simulink model "Multibody_model_El_winch"  (R2023b)
settings: Solver=FixedStepAuto  StartTime=0.0  StopTime=25  FixedStep=0.001  RelTol=1e-3
model workspace (MATLAB code in the model file):
  | % Parameters
  | Q_max = 130; %L/min |  2 vales w max 65 L/min
  | 
  | %Load Parameters
  | m_pl = 1000;
  | r_d = 0.035;
  | ig = 5;
  | J_drum = 0.0006125; % 1/2MR^2
  | b_hat = 0.001;
  | 
  | % Motor Parameters
  | np=2;
  | P_N = 15000;
  | n_eff = 0.917;
  | n_rpm = 1469;
  | pf = 0.84;
  | I_N = 29;
  | Is_In = 8;
  | T_n = 97.5;
  | Ti_Tn = 3.1;
  | Tb_Tn = 3.6;
  | J_motor = 0.13;
  | 
  | % Inv-Gamma Circuit parameters
  | 
  | R_R_hat = 0.2052;
  | X_M_opt = 15.1061;
  | X_sig_opt = 0.3774;
  | omega_rN = 307.6666;
  | omega_N = 314.1593;
  | omega1 = omega_rN;
  | L_M_hat = X_M_opt/omega1;
  | L_sig_hat = X_sig_opt/omega1;
  | R_s = 0.619;
  | 
  | 
  | psi_ref = 20*P_N/(sqrt(2)*pi*np*I_N*n_rpm);
  | 
  | % Others
  | V_base = 400*sqrt(2)/sqrt(3);
  | I_max = I_N*3;
  | 
  | % Speed Controller
  | t_r = 1e-3;
  | w_BW = log(9)/t_r;
  | w_BWs = 0.1*w_BW;
  | J_hat = m_pl*((r_d/(ig))^2) + J_drum*((1/ig)^2) + J_motor;
  | kps = 2*J_hat*w_BWs/(3*np^2*psi_ref);
  | kis = w_BWs^2*2*J_hat/(3*np^2*psi_ref);
  | Ba = 2*J_hat/(3*np^2*psi_ref)*(w_BWs-b_hat/J_hat);
  | 
  | % Current Controller
  | kp = w_BW*L_sig_hat;
  | ki = w_BW^2*L_sig_hat;
  | Ra = w_BW*L_sig_hat - (R_R_hat + R_s);
  | R = R_R_hat + R_s;
undefined symbols (not defined in the file or in its folder): j, magnitude, X, Y, Z
libraries: sm_lib x44, fl_lib x24, nesl_utility x22, SimscapeFluids_lib x8, slpidlib x4, spsRMSLib x1, simulink x1
(part 3 of 4)

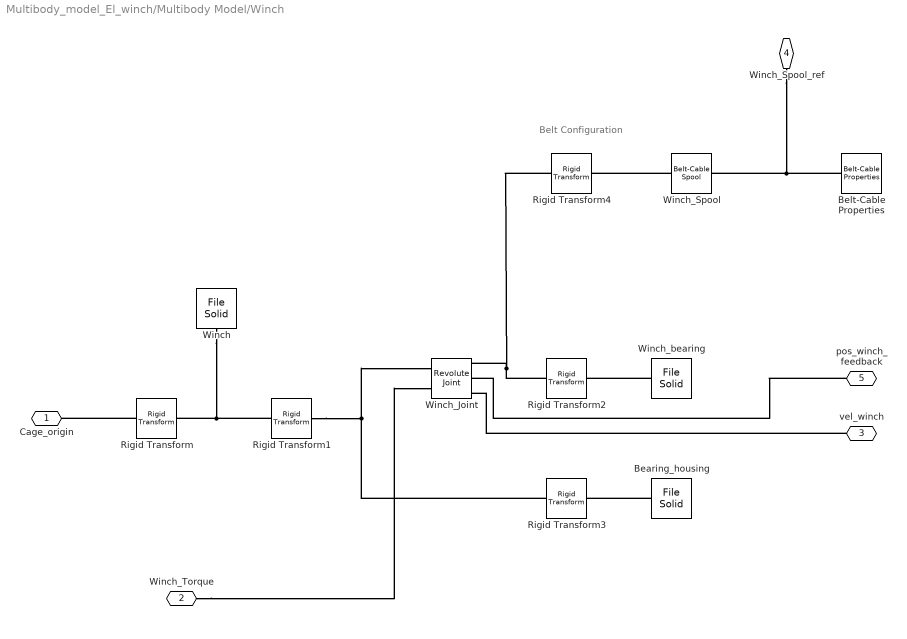
== system Multibody_model_El_winch/Multibody Model/Winch ==
  note: Belt Configuration
  Bearing_housing : sm_lib/Body Elements/File Solid  ExtGeomFileName=.\Parts_and_stl\Frame_connection_winch.STL  UnitType=Custom  ExtGeomFileUnits=mm  StepReaderType=HEX  ExportConvexHullGeometry=off  InertiaType=Custom  Mass=1  MassUnits=kg  CenterOfMass=[0 0 0]  CenterOfMassUnits=m  MomentsOfInertia=[1 1 1]  MomentsOfInertiaUnits=kg*m^2  ProductsOfInertia=[0 0 0]  ProductsOfInertiaUnits=kg*m^2  BasedOnType=DensityFromFile  Density=1000  DensityUnits=kg/m^3  DoExposeReferenceFrame=on  SerializedFrames=<Frames/>  GraphicType=FromGeometry  MarkerShape=Sphere  MarkerSize=10  GraphicVisPropType=SimpleVisualProperties  GraphicDiffuseColor=[0.0 0.0 0.0]  GraphicSpecularColor=[0.5 0.5 0.5 1.0]  GraphicAmbientColor=[0.15 0.15 0.15 1.0]  GraphicEmissiveColor=[0.0 0.0 0.0 1.0]  GraphicShininess=75  GraphicOpacity=1.0
  Belt-Cable Properties : sm_lib/Belts and Cables/Belt-Cable Properties  DrumBeltCableAlignment=Unrestricted  GraphicType=PitchLine  GraphicVisPropType=SimpleVisualProperties  GraphicDiffuseColor=[0.5 0.5 0.5]  GraphicSpecularColor=[0.5 0.5 0.5 1.0]  GraphicAmbientColor=[0.15 0.15 0.15 1.0]  GraphicEmissiveColor=[0.0 0.0 0.0 1.0]  GraphicShininess=75  GraphicOpacity=1.0
  Rigid Transform : sm_lib/Frames and Transforms/Rigid Transform  TranslationMethod=Cartesian  TranslationStandardOffset=0  TranslationStandardOffsetUnits=m  TranslationStandardAxis=+Z  TranslationCartesianOffset=[2296 1499.2 513]  TranslationCartesianOffsetUnits=mm  TranslationROffset=0  TranslationROffsetUnits=m  TranslationZOffset=0  TranslationZOffsetUnits=m  TranslationThetaOffset=0  TranslationThetaOffsetUnits=deg  RotationMethod=RotationSequence  RotationAngleUnits=deg  RotationStandardAxis=+Z  RotationAngle=0.0  RotationArbitraryAxis=[0 0 1]  FollAlignAxisA=+X  BaseAlignAxisA=+Y  FollAlignAxisB=+Y  BaseAlignAxisB=+Z  RotationSequenceAxes=FollowerAxes  RotationSequence=XYZ  RotationSequenceAngles=[-90 0 180]  RotationSequenceAnglesUnits=deg  RotationMatrix=[1 0 0; 0 1 0; 0 0 1]  Quaternion=[1 0 0 0]
  Rigid Transform1 : sm_lib/Frames and Transforms/Rigid Transform  TranslationMethod=Cartesian  TranslationStandardOffset=0  TranslationStandardOffsetUnits=m  TranslationStandardAxis=+Z  TranslationCartesianOffset=[-100 -74.50 180.818]  TranslationCartesianOffsetUnits=mm  TranslationROffset=0  TranslationROffsetUnits=m  TranslationZOffset=0  TranslationZOffsetUnits=m  TranslationThetaOffset=0  TranslationThetaOffsetUnits=deg  RotationMethod=RotationSequence  RotationAngleUnits=deg  RotationStandardAxis=+Z  RotationAngle=0.0  RotationArbitraryAxis=[0 0 1]  FollAlignAxisA=+X  BaseAlignAxisA=+Y  FollAlignAxisB=+Y  BaseAlignAxisB=+Z  RotationSequenceAxes=FollowerAxes  RotationSequence=XYZ  RotationSequenceAngles=[90 0 0]  RotationSequenceAnglesUnits=deg  RotationMatrix=[1 0 0; 0 1 0; 0 0 1]  Quaternion=[1 0 0 0]
  Rigid Transform2 : sm_lib/Frames and Transforms/Rigid Transform  TranslationMethod=Cartesian  TranslationStandardOffset=0  TranslationStandardOffsetUnits=m  TranslationStandardAxis=+Z  TranslationCartesianOffset=[0 0 -80]  TranslationCartesianOffsetUnits=mm  TranslationROffset=0  TranslationROffsetUnits=m  TranslationZOffset=0  TranslationZOffsetUnits=m  TranslationThetaOffset=0  TranslationThetaOffsetUnits=deg  RotationMethod=None  RotationAngleUnits=deg  RotationStandardAxis=+Z  RotationAngle=0.0  RotationArbitraryAxis=[0 0 1]  FollAlignAxisA=+X  BaseAlignAxisA=+Y  FollAlignAxisB=+Y  BaseAlignAxisB=+Z  RotationSequenceAxes=FollowerAxes  RotationSequence=XYX  RotationSequenceAngles=[0 0 0]  RotationSequenceAnglesUnits=deg  RotationMatrix=[1 0 0; 0 1 0; 0 0 1]  Quaternion=[1 0 0 0]
  Rigid Transform3 : sm_lib/Frames and Transforms/Rigid Transform  TranslationMethod=Cartesian  TranslationStandardOffset=0  TranslationStandardOffsetUnits=m  TranslationStandardAxis=+Z  TranslationCartesianOffset=[0 0 207]  TranslationCartesianOffsetUnits=mm  TranslationROffset=0  TranslationROffsetUnits=m  TranslationZOffset=0  TranslationZOffsetUnits=m  TranslationThetaOffset=0  TranslationThetaOffsetUnits=deg  RotationMethod=RotationSequence  RotationAngleUnits=deg  RotationStandardAxis=+Z  RotationAngle=0.0  RotationArbitraryAxis=[0 0 1]  FollAlignAxisA=+X  BaseAlignAxisA=+Y  FollAlignAxisB=+Y  BaseAlignAxisB=+Z  RotationSequenceAxes=FollowerAxes  RotationSequence=XYZ  RotationSequenceAngles=[90 0 0]  RotationSequenceAnglesUnits=deg  RotationMatrix=[1 0 0; 0 1 0; 0 0 1]  Quaternion=[1 0 0 0]
  Rigid Transform4 : sm_lib/Frames and Transforms/Rigid Transform  TranslationMethod=Cartesian  TranslationStandardOffset=0  TranslationStandardOffsetUnits=m  TranslationStandardAxis=+Z  TranslationCartesianOffset=[0 0 130]  TranslationCartesianOffsetUnits=mm  TranslationROffset=0  TranslationROffsetUnits=m  TranslationZOffset=0  TranslationZOffsetUnits=m  TranslationThetaOffset=0  TranslationThetaOffsetUnits=deg  RotationMethod=None  RotationAngleUnits=deg  RotationStandardAxis=+Z  RotationAngle=0.0  RotationArbitraryAxis=[0 0 1]  FollAlignAxisA=+X  BaseAlignAxisA=+Y  FollAlignAxisB=+Y  BaseAlignAxisB=+Z  RotationSequenceAxes=FollowerAxes  RotationSequence=XYX  RotationSequenceAngles=[0 0 0]  RotationSequenceAnglesUnits=deg  RotationMatrix=[1 0 0; 0 1 0; 0 0 1]  Quaternion=[1 0 0 0]
  Winch : sm_lib/Body Elements/File Solid  ExtGeomFileName=.\Parts_and_stl\Winch.STL  UnitType=Custom  ExtGeomFileUnits=mm  StepReaderType=HEX  ExportConvexHullGeometry=off  InertiaType=Custom  Mass=1  MassUnits=kg  CenterOfMass=[0 0 0]  CenterOfMassUnits=m  MomentsOfInertia=[1 1 1]  MomentsOfInertiaUnits=kg*m^2  ProductsOfInertia=[0 0 0]  ProductsOfInertiaUnits=kg*m^2  BasedOnType=DensityFromFile  Density=1000  DensityUnits=kg/m^3  DoExposeReferenceFrame=on  SerializedFrames=<Frames/>  GraphicType=FromGeometry  MarkerShape=Sphere  MarkerSize=10  GraphicVisPropType=SimpleVisualProperties  GraphicDiffuseColor=[1.0 0.0 0.2]  GraphicSpecularColor=[0.5 0.5 0.5 1.0]  GraphicAmbientColor=[0.15 0.15 0.15 1.0]  GraphicEmissiveColor=[0.0 0.0 0.0 1.0]  GraphicShininess=75  GraphicOpacity=1.0
  Winch_Joint : sm_lib/Joints/Revolute Joint  JointMode=Normal  SenseConstraintForce=off  SenseConstraintForceX=off  SenseConstraintForceY=off  SenseConstraintForceZ=off  SenseConstraintTorque=off  SenseConstraintTorqueX=off  SenseConstraintTorqueY=off  SenseConstraintTorqueZ=off  SenseTotalForce=off  SenseTotalForceX=off  SenseTotalForceY=off  SenseTotalForceZ=off  SenseTotalTorque=off  SenseTotalTorqueX=off  SenseTotalTorqueY=off  SenseTotalTorqueZ=off  CompositeWrenchDir=FollowerOnBase  CompositeWrenchFrame=BaseFrame  EquilibriumPosition=0  EquilibriumPositionUnits=deg  SpringStiffness=0  SpringStiffnessUnits=N*m/deg  DampingCoefficient=0  DampingCoefficientUnits=N*m/(deg/s)  TorqueActuationMode=InputTorque  MotionActuationMode=ComputedMotion  SensePosition=on  SenseVelocity=on  SenseAcceleration=off  SenseTorqueForce=off  SenseLowerLimitTorqueForce=off  SenseUpperLimitTorqueForce=off  LowerLimitSpecify=off  LowerLimitBound=-90  LowerLimitBoundUnits=deg  LowerLimitStiffness=1e4  LowerLimitStiffnessUnits=N*m/deg  LowerLimitDamping=10  LowerLimitDampingUnits=N*m/(deg/s)  LowerLimitTransitionRegionWidth=0.1  LowerLimitTransitionRegionWidthUnits=deg  UpperLimitSpecify=off  UpperLimitBound=90  UpperLimitBoundUnits=deg  UpperLimitStiffness=1e4  UpperLimitStiffnessUnits=N*m/deg  UpperLimitDamping=10  UpperLimitDampingUnits=N*m/(deg/s)  UpperLimitTransitionRegionWidth=0.1  UpperLimitTransitionRegionWidthUnits=deg  PositionTargetSpecify=off  PositionTargetPriority=High  PositionTargetValue=7  PositionTargetValueUnits=deg  VelocityTargetSpecify=off  VelocityTargetPriority=High  VelocityTargetValue=0  VelocityTargetValueUnits=deg/s
  Winch_Spool : sm_lib/Belts and Cables/Belt-Cable Spool  PitchRadius=70/2  PitchRadiusUnits=mm  SenseSpoolAngleA=off  SenseFleetAngleA=off
  Winch_bearing : sm_lib/Body Elements/File Solid  ExtGeomFileName=.\Parts_and_stl\Winch_revolute_pin.STL  UnitType=Custom  ExtGeomFileUnits=mm  StepReaderType=HEX  ExportConvexHullGeometry=off  InertiaType=Custom  Mass=1  MassUnits=kg  CenterOfMass=[0 0 0]  CenterOfMassUnits=m  MomentsOfInertia=[1 1 1]  MomentsOfInertiaUnits=kg*m^2  ProductsOfInertia=[0 0 0]  ProductsOfInertiaUnits=kg*m^2  BasedOnType=DensityFromFile  Density=1000  DensityUnits=kg/m^3  DoExposeReferenceFrame=on  SerializedFrames=<Frames/>  GraphicType=FromGeometry  MarkerShape=Sphere  MarkerSize=10  GraphicVisPropType=SimpleVisualProperties  GraphicDiffuseColor=[0.0 0.8 0.0]  GraphicSpecularColor=[0.5 0.5 0.5 1.0]  GraphicAmbientColor=[0.15 0.15 0.15 1.0]  GraphicEmissiveColor=[0.0 0.0 0.0 1.0]  GraphicShininess=75  GraphicOpacity=1.0
  Cage_origin : PMIOPort  Side=Left
  Winch_Torque : PMIOPort  Port=2  Side=Right
  vel_winch : PMIOPort  Port=3  Side=Right
  Winch_Spool_ref : PMIOPort  Port=4  Side=Right
  pos_winch_feedback : PMIOPort  Port=5  Side=Left
  connections:
  Winch/RConn1 -- Rigid Transform1/LConn1 -- Rigid Transform/RConn1
  Rigid Transform1/RConn1 -- Rigid Transform3/LConn1 -- Winch_Joint/LConn1
  Winch_bearing/RConn1 -- Rigid Transform2/RConn1
  Bearing_housing/RConn1 -- Rigid Transform3/RConn1
  Rigid Transform/LConn1 -- Cage_origin/RConn1
  Rigid Transform2/LConn1 -- Rigid Transform4/LConn1 -- Winch_Joint/RConn1
  Winch_Spool/LConn1 -- Rigid Transform4/RConn1
  Belt-Cable Properties/LConn1 -- Winch_Spool_ref/RConn1 -- Winch_Spool/RConn1
  vel_winch/RConn1 -- Winch_Joint/RConn3
  pos_winch_feedback/RConn1 -- Winch_Joint/RConn2
  Winch_Torque/RConn1 -- Winch_Joint/LConn2

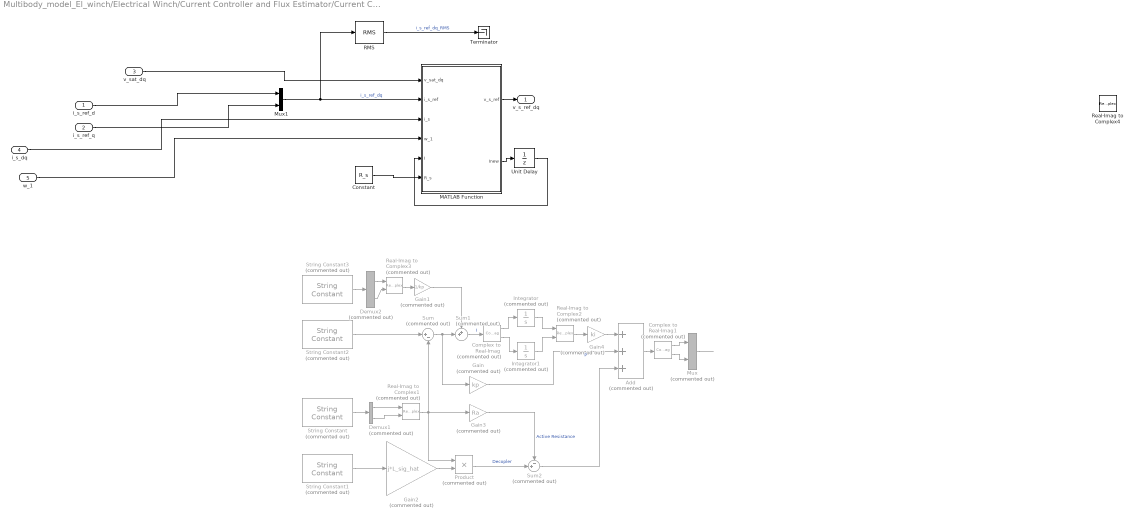
== system Multibody_model_El_winch/Electrical Winch/Current Controller and Flux Estimator/Current Controller ==
  i_s_ref_d : Inport
  i_s_ref_q : Inport  Port=2
  v_sat_dq : Inport  Port=3
  i_s_dq : Inport  Port=4
  w_1 : Inport  Port=5
  Add : Sum  Commented=on  Inputs=+++
  Complex to Real-Imag : ComplexToRealImag  Commented=on
  Complex to Real-Imag1 : ComplexToRealImag  Commented=on
  Constant : Constant  Value=R_s
  Demux1 : Demux  Commented=on  Outputs=2
  Demux2 : Demux  Commented=on  Outputs=2
  Gain : Gain  Commented=on  Gain=kp
  Gain1 : Gain  Commented=on  Gain=1/kp
  Gain2 : Gain  Commented=on  Gain=j*L_sig_hat
  Gain3 : Gain  Commented=on  Gain=Ra
  Gain4 : Gain  Commented=on  Gain=ki
  Integrator : Integrator  Commented=on
  Integrator1 : Integrator  Commented=on
  MATLAB Function : MATLAB Function  TreatAsAtomicUnit=on
  Mux : Mux  Commented=on  Inputs=2
  Mux1 : Mux  Inputs=2
  Product : Product  Commented=on
  RMS : spsRMSLib/RMS  TrueRMS=on  Freq=60  RMSInit=120  Ts=0
  Real-Imag to Complex1 : RealImagToComplex  Commented=on
  Real-Imag to Complex2 : RealImagToComplex  Commented=on
  Real-Imag to Complex3 : RealImagToComplex  Commented=on
  Real-Imag to Complex4 : RealImagToComplex
  String Constant : StringConstant  Commented=on  String=i_s_dq
  String Constant1 : StringConstant  Commented=on  String=w_1
  String Constant2 : StringConstant  Commented=on  String=i_s_ref_dq
  String Constant3 : StringConstant  Commented=on  String=v_sat_dq
  Sum : Sum  Commented=on  Inputs=|+-
  Sum1 : Sum  Commented=on  Inputs=++|
  Sum2 : Sum  Commented=on  Inputs=-+|
  Terminator : Terminator
  Unit Delay : UnitDelay  SampleTime=-1  HasFrameUpgradeWarning=on
  v_s_ref_dq : Outport  PortDimensions=2
  wires:
  MATLAB Function/2(Inew) -> Unit Delay/1
  Mux1/1 -> RMS/1, MATLAB Function/2(i_s_ref)  "i_s_ref_dq"
  w_1/1 -> MATLAB Function/4(w_1)
  i_s_dq/1 -> MATLAB Function/3(i_s)
  Unit Delay/1 -> MATLAB Function/5(I)
  MATLAB Function/1(v_s_ref) -> v_s_ref_dq/1
  v_sat_dq/1 -> MATLAB Function/1(v_sat_dq)
  Constant/1 -> MATLAB Function/6(R_s)
  String Constant2/1 -> Sum/1
  Demux1/2 -> Real-Imag to Complex1/2
  Demux1/1 -> Real-Imag to Complex1/1
  Real-Imag to Complex1/1 -> Gain3/1, Product/1, Sum/2
  Sum/1 -> Sum1/2, Gain/1
  Sum1/1 -> Complex to Real-Imag/1  "I"
  Complex to Real-Imag/2 -> Integrator1/1
  Complex to Real-Imag/1 -> Integrator/1
  Integrator/1 -> Real-Imag to Complex2/1
  Integrator1/1 -> Real-Imag to Complex2/2
  Gain1/1 -> Sum1/1
  Gain2/1 -> Product/2
  Real-Imag to Complex2/1 -> Gain4/1
  Add/1 -> Complex to Real-Imag1/1
  Complex to Real-Imag1/2 -> Mux/2
  Complex to Real-Imag1/1 -> Mux/1
  Demux2/2 -> Real-Imag to Complex3/2
  Demux2/1 -> Real-Imag to Complex3/1
  Product/1 -> Sum2/2  "Decopler"
  Gain3/1 -> Sum2/1  "Active Resistance"
  Sum2/1 -> Add/3
  Gain4/1 -> Add/1
  Gain/1 -> Add/2  "P"
  Real-Imag to Complex3/1 -> Gain1/1
  i_s_ref_d/1 -> Mux1/1
  i_s_ref_q/1 -> Mux1/2
  RMS/1 -> Terminator/1  "i_s_ref_dq_RMS"
  String Constant/1 -> Demux1/1
  String Constant1/1 -> Gain2/1
  String Constant3/1 -> Demux2/1
  Mux/1 -> ?

== system Multibody_model_El_winch/Electrical Winch/Current Controller and Flux Estimator/FeedFWD ==
  v_s_ref_dq : Inport
  psi_r : Inport  Port=2
  Constant : Constant  Value=R_R_hat/L_M_hat * psi_ref
  Demux : Demux  Outputs=2
  Mux : Mux  Inputs=2
  Sum : Sum  Inputs=-+|
  Sum1 : Sum  Inputs=|++
  v_dq_ref : Outport
  wires:
  v_s_ref_dq/1 -> Demux/1
  Mux/1 -> v_dq_ref/1
  Sum/1 -> Mux/1
  Demux/1 -> Sum/2
  Constant/1 -> Sum/1
  Demux/2 -> Sum1/1
  Sum1/1 -> Mux/2
  psi_r/1 -> Sum1/2

== system Multibody_model_El_winch/Electrical Winch/Current Controller and Flux Estimator/Flux Estimator ==
  note: Initial condition: psi_ref
  i_dq_ref : Inport
  w_r : Inport  Port=2
  Demux1 : Demux  Outputs=2
  Gain : Gain  Gain=1/L_M_hat
  Gain1 : Gain  Gain=R_R_hat
  Gain2 : Gain  Gain=R_R_hat
  Integrator : Integrator  InitialCondition=psi_ref
  Product : Product  Inputs=/*
  Sum : Sum  Inputs=|+-
  Sum1 : Sum  Inputs=|++
  w_1 : Outport
  psi_r : Outport  Port=2
  wires:
  Product/1 -> Gain2/1
  Demux1/2 -> Product/2
  Gain1/1 -> Integrator/1
  Sum/1 -> Gain1/1
  Gain/1 -> Sum/2
  Integrator/1 -> Gain/1, psi_r/1, Product/1
  i_dq_ref/1 -> Demux1/1
  Demux1/1 -> Sum/1
  w_r/1 -> Sum1/2
  Gain2/1 -> Sum1/1
  Sum1/1 -> w_1/1

== system Multibody_model_El_winch/Electrical Winch/Current Controller and Flux Estimator/IM ==
  vs_abc : Inport
  w_m : Inport  Port=2
  Electromagnetic Torque : Subsystem
  Flux Equations : Subsystem
  Gain : Gain  Gain=np  SaturateOnIntegerOverflow=on  OutDataTypeStr=Inherit: Same as input  ParamDataTypeStr=Inherit: Same as input
  Voltage Equations : Subsystem
  abc->alphabeta : Subsystem
  alphabeta->abc : Subsystem
  is_abc : Outport
  T_em : Outport  Port=2
  wires:
  Gain/1 -> Voltage Equations/3(w_r)
  alphabeta->abc/1(is_abc) -> is_abc/1
  abc->alphabeta/1(v_s^s) -> Voltage Equations/1(v_s^s)
  Voltage Equations/1(psi_s^s) -> Flux Equations/1(psi_s^s)
  Voltage Equations/2(psi_R^s) -> Flux Equations/2(psi_R^s), Electromagnetic Torque/2(psi_R^s)
  vs_abc/1 -> abc->alphabeta/1(vs_abc)
  Flux Equations/1(i_s^s) -> Electromagnetic Torque/1(i_s^s), Voltage Equations/2(i_s^s), alphabeta->abc/1(i_s^s)
  Electromagnetic Torque/1(T_em) -> T_em/1
  w_m/1 -> Gain/1
  Flux Equations/2(i_R^s) -> Voltage Equations/4(i_R^s)

== system Multibody_model_El_winch/Electrical Winch/Current Controller and Flux Estimator/Id_ref ==
  v_dq_ref : Inport
  omega_1 : Inport  Port=2
  Abs : Abs  SaturateOnIntegerOverflow=off
  Constant : Constant  Value=V_base^2
  Constant2 : Constant  Value=2*pi*50
  Demux : Demux  Outputs=2
  Limits : Integrator  InitialCondition=psi_ref/L_M_hat  LimitOutput=on  UpperSaturationLimit=psi_ref/L_M_hat  LowerSaturationLimit=0.1*psi_ref/L_M_hat
  Math Function : Math  Operator=magnitude^2
  Math Function1 : Math  Operator=magnitude^2
  Max : MinMax  Function=max  Inputs=2
  Product : Product  Inputs=*/
  Sum : Sum  Inputs=-+-
  k_fw : Gain  Gain=R_R_hat/((L_sig_hat^2)*V_base)
  i_d_ref : Outport
  wires:
  Demux/2 -> Math Function1/1  "v_q"
  Sum/1 -> k_fw/1
  Math Function1/1 -> Sum/3
  Math Function/1 -> Sum/1
  Limits/1 -> i_d_ref/1
  v_dq_ref/1 -> Demux/1
  Demux/1 -> Math Function/1  "v_d"
  Product/1 -> Limits/1
  Constant/1 -> Sum/2
  k_fw/1 -> Product/1
  Max/1 -> Product/2
  Constant2/1 -> Max/2  "nominal rotor speed"
  Abs/1 -> Max/1
  omega_1/1 -> Abs/1  "rotor speed"

== system Multibody_model_El_winch/Electrical Winch/Current Controller and Flux Estimator/abc->dq1 ==
  is_abc : Inport
  thetas : Inport  Port=2
  MATLAB Function : MATLAB Function  TreatAsAtomicUnit=on
  Scope : Scope
  is_dq : Outport
  wires:
  thetas/1 -> MATLAB Function/2(thetas)
  is_abc/1 -> MATLAB Function/1(is_abc)
  MATLAB Function/1(is) -> Scope/1, is_dq/1

== system Multibody_model_El_winch/Electrical Winch/Current Controller and Flux Estimator/dq->abc ==
  vs_dq : Inport
  thetas : Inport  Port=2
  MATLAB Function : MATLAB Function  TreatAsAtomicUnit=on
  Scope : Scope
  vs_abc : Outport
  wires:
  vs_dq/1 -> MATLAB Function/1(vs_dq)
  thetas/1 -> MATLAB Function/2(thetas)
  MATLAB Function/1(vs_abc) -> Scope/1, vs_abc/1

== system Multibody_model_El_winch/Electrical Winch/Current Controller and Flux Estimator/saturation ==
  v_s_ref_dq : Inport
  Complex to Magnitude-Angle : ComplexToMagnitudeAngle
  Complex to Real-Imag : ComplexToRealImag
  Demux1 : Demux  Outputs=2
  Magnitude-Angle to Complex : MagnitudeAngleToComplex
  Mux1 : Mux  Inputs=2
  Real-Imag to Complex : RealImagToComplex
  Saturation : Saturate  UpperLimit=400*sqrt(2)*sqrt(3)  LowerLimit=0
  vs_dq : Outport
  wires:
  Mux1/1 -> vs_dq/1
  Demux1/2 -> Real-Imag to Complex/2
  Complex to Real-Imag/1 -> Mux1/1
  Magnitude-Angle to Complex/1 -> Complex to Real-Imag/1
  Demux1/1 -> Real-Imag to Complex/1
  Real-Imag to Complex/1 -> Complex to Magnitude-Angle/1
  Complex to Real-Imag/2 -> Mux1/2
  v_s_ref_dq/1 -> Demux1/1
  Complex to Magnitude-Angle/1 -> Saturation/1
  Saturation/1 -> Magnitude-Angle to Complex/1  "sat"
  Complex to Magnitude-Angle/2 -> Magnitude-Angle to Complex/2

== system Multibody_model_El_winch/Hydraulic System/Cont_pressure_source/V_0 ==
  Constant Volume Chamber (IL) : fl_lib/Isothermal Liquid/Elements/Constant Volume Chamber (IL)  volume=1 l  p_I_specify=off  p_I_priority=High  p_I=0.101325 MPa  p_I_nominal_specify=off  p_I_nominal_unit=MPa  p_I_nominal_value=1
      settings: InternalSimscapePortConfiguration="{\"Bottom\":[],\"Left\":[{\"id\":\"A\",\"label\":\"A\",\"type\":\"foundation.isothermal_liquid.isothermal_liquid\"}],\"Right\":[],\"Top\":[]}"
  Gain : Gain  Gain=1/10^5
  PS-Simulink Converter : nesl_utility/PS-Simulink Converter  PhysicalDomain=network_engine_domain  SubClassName=ps_output  LeftPortType=input  RightPortType=output  PseudoPeriodic=off  Frequencies=[]  VectorFormat=inherit  Unit=inherit  AffineConversion=off
  Pressure Sensor (IL) : fl_lib/Isothermal Liquid/Sensors/Pressure Sensor (IL)  pressure_measure=foundation.enum.pressure_measure.gauge
      settings: InternalSimscapePortConfiguration="{\"Bottom\":[],\"Left\":[{\"id\":\"A\",\"label\":\"A\",\"type\":\"foundation.isothermal_liquid.isothermal_liquid\"}],\"Right\":[{\"id\":\"Pg\",\"label\":\"Pg\",\"type\":\"output\"}],\"Top\":[]}"
  Connection Port : PMIOPort  Side=Left
  Out1 : Outport
  wires:
  Gain/1 -> Out1/1
  PS-Simulink Converter/1 -> Gain/1
  connections:
  Pressure Sensor (IL)/LConn1 -- Constant Volume Chamber (IL)/LConn1 -- Connection Port/RConn1
  PS-Simulink Converter/LConn1 -- Pressure Sensor (IL)/RConn1

== system Multibody_model_El_winch/Hydraulic System/DCV_cylinder/QM_0 ==
  Flow Rate Sensor (IL) : fl_lib/Isothermal Liquid/Sensors/Flow Rate Sensor (IL)  sensor_type=foundation.enum.mass_volumetric_sensor.volumetric
      settings: InternalSimscapePortConfiguration="{\"Bottom\":[],\"Left\":[{\"id\":\"A\",\"label\":\"A\",\"type\":\"foundation.isothermal_liquid.isothermal_liquid\"}],\"Right\":[{\"id\":\"B\",\"label\":\"B\",\"type\":\"foundation.isothermal_liquid.isothermal_liquid\"},{\"id\":\"V\",\"label\":\"V\",\"type\":\"output\"}],\"Top\":[]}"
  Gain : Gain  Gain=6e4
  PS-Simulink Converter : nesl_utility/PS-Simulink Converter  PhysicalDomain=network_engine_domain  SubClassName=ps_output  LeftPortType=input  RightPortType=output  PseudoPeriodic=off  Frequencies=[]  VectorFormat=inherit  Unit=inherit  AffineConversion=off
  A : PMIOPort  Side=Left
  B : PMIOPort  Port=2  Side=Right
  Q : Outport
  wires:
  PS-Simulink Converter/1 -> Gain/1
  Gain/1 -> Q/1
  connections:
  PS-Simulink Converter/LConn1 -- Flow Rate Sensor (IL)/RConn2
  A/RConn1 -- Flow Rate Sensor (IL)/LConn1
  B/RConn1 -- Flow Rate Sensor (IL)/RConn1

== system Multibody_model_El_winch/Hydraulic System/DCV_cylinder/QM_1 ==
  Flow Rate Sensor (IL) : fl_lib/Isothermal Liquid/Sensors/Flow Rate Sensor (IL)  sensor_type=foundation.enum.mass_volumetric_sensor.volumetric
      settings: InternalSimscapePortConfiguration="{\"Bottom\":[],\"Left\":[{\"id\":\"A\",\"label\":\"A\",\"type\":\"foundation.isothermal_liquid.isothermal_liquid\"}],\"Right\":[{\"id\":\"B\",\"label\":\"B\",\"type\":\"foundation.isothermal_liquid.isothermal_liquid\"},{\"id\":\"V\",\"label\":\"V\",\"type\":\"output\"}],\"Top\":[]}"
  Gain : Gain  Gain=6e4
  PS-Simulink Converter : nesl_utility/PS-Simulink Converter  PhysicalDomain=network_engine_domain  SubClassName=ps_output  LeftPortType=input  RightPortType=output  PseudoPeriodic=off  Frequencies=[]  VectorFormat=inherit  Unit=inherit  AffineConversion=off
  A : PMIOPort  Side=Left
  B : PMIOPort  Port=2  Side=Right
  Q : Outport
  wires:
  PS-Simulink Converter/1 -> Gain/1
  Gain/1 -> Q/1
  connections:
  PS-Simulink Converter/LConn1 -- Flow Rate Sensor (IL)/RConn2
  A/RConn1 -- Flow Rate Sensor (IL)/LConn1
  B/RConn1 -- Flow Rate Sensor (IL)/RConn1

== system Multibody_model_El_winch/Hydraulic System/DCV_cylinder/V_A ==
  Constant Volume Chamber (IL) : fl_lib/Isothermal Liquid/Elements/Constant Volume Chamber (IL)  volume=1 l  p_I_specify=off  p_I_priority=High  p_I=0.101325 MPa  p_I_nominal_specify=off  p_I_nominal_unit=MPa  p_I_nominal_value=1
      settings: InternalSimscapePortConfiguration="{\"Bottom\":[],\"Left\":[{\"id\":\"A\",\"label\":\"A\",\"type\":\"foundation.isothermal_liquid.isothermal_liquid\"}],\"Right\":[],\"Top\":[]}"
  Gain : Gain  Gain=1/10^5
  PS-Simulink Converter : nesl_utility/PS-Simulink Converter  PhysicalDomain=network_engine_domain  SubClassName=ps_output  LeftPortType=input  RightPortType=output  PseudoPeriodic=off  Frequencies=[]  VectorFormat=inherit  Unit=inherit  AffineConversion=off
  Pressure Sensor (IL) : fl_lib/Isothermal Liquid/Sensors/Pressure Sensor (IL)  pressure_measure=foundation.enum.pressure_measure.gauge
      settings: InternalSimscapePortConfiguration="{\"Bottom\":[],\"Left\":[{\"id\":\"A\",\"label\":\"A\",\"type\":\"foundation.isothermal_liquid.isothermal_liquid\"}],\"Right\":[{\"id\":\"Pg\",\"label\":\"Pg\",\"type\":\"output\"}],\"Top\":[]}"
  Connection Port : PMIOPort  Side=Left
  Out1 : Outport
  wires:
  Gain/1 -> Out1/1
  PS-Simulink Converter/1 -> Gain/1
  connections:
  Pressure Sensor (IL)/LConn1 -- Constant Volume Chamber (IL)/LConn1 -- Connection Port/RConn1
  PS-Simulink Converter/LConn1 -- Pressure Sensor (IL)/RConn1

== system Multibody_model_El_winch/Hydraulic System/DCV_cylinder/V_B ==
  Constant Volume Chamber (IL) : fl_lib/Isothermal Liquid/Elements/Constant Volume Chamber (IL)  volume=1 l  p_I_specify=off  p_I_priority=High  p_I=0.101325 MPa  p_I_nominal_specify=off  p_I_nominal_unit=MPa  p_I_nominal_value=1
      settings: InternalSimscapePortConfiguration="{\"Bottom\":[],\"Left\":[{\"id\":\"A\",\"label\":\"A\",\"type\":\"foundation.isothermal_liquid.isothermal_liquid\"}],\"Right\":[],\"Top\":[]}"
  Gain : Gain  Gain=1/10^5
  PS-Simulink Converter : nesl_utility/PS-Simulink Converter  PhysicalDomain=network_engine_domain  SubClassName=ps_output  LeftPortType=input  RightPortType=output  PseudoPeriodic=off  Frequencies=[]  VectorFormat=inherit  Unit=inherit  AffineConversion=off
  Pressure Sensor (IL) : fl_lib/Isothermal Liquid/Sensors/Pressure Sensor (IL)  pressure_measure=foundation.enum.pressure_measure.gauge
      settings: InternalSimscapePortConfiguration="{\"Bottom\":[],\"Left\":[{\"id\":\"A\",\"label\":\"A\",\"type\":\"foundation.isothermal_liquid.isothermal_liquid\"}],\"Right\":[{\"id\":\"Pg\",\"label\":\"Pg\",\"type\":\"output\"}],\"Top\":[]}"
  Connection Port : PMIOPort  Side=Left
  Out1 : Outport
  wires:
  Gain/1 -> Out1/1
  PS-Simulink Converter/1 -> Gain/1
  connections:
  Pressure Sensor (IL)/LConn1 -- Constant Volume Chamber (IL)/LConn1 -- Connection Port/RConn1
  PS-Simulink Converter/LConn1 -- Pressure Sensor (IL)/RConn1

== system Multibody_model_El_winch/Hydraulic System/DCV_cylinder/V_in ==
  Constant Volume Chamber (IL) : fl_lib/Isothermal Liquid/Elements/Constant Volume Chamber (IL)  volume=1 l  p_I_specify=off  p_I_priority=High  p_I=0.101325 MPa  p_I_nominal_specify=off  p_I_nominal_unit=MPa  p_I_nominal_value=1
      settings: InternalSimscapePortConfiguration="{\"Bottom\":[],\"Left\":[{\"id\":\"A\",\"label\":\"A\",\"type\":\"foundation.isothermal_liquid.isothermal_liquid\"}],\"Right\":[],\"Top\":[]}"
  Gain : Gain  Gain=1/10^5
  PS-Simulink Converter : nesl_utility/PS-Simulink Converter  PhysicalDomain=network_engine_domain  SubClassName=ps_output  LeftPortType=input  RightPortType=output  PseudoPeriodic=off  Frequencies=[]  VectorFormat=inherit  Unit=inherit  AffineConversion=off
  Pressure Sensor (IL) : fl_lib/Isothermal Liquid/Sensors/Pressure Sensor (IL)  pressure_measure=foundation.enum.pressure_measure.gauge
      settings: InternalSimscapePortConfiguration="{\"Bottom\":[],\"Left\":[{\"id\":\"A\",\"label\":\"A\",\"type\":\"foundation.isothermal_liquid.isothermal_liquid\"}],\"Right\":[{\"id\":\"Pg\",\"label\":\"Pg\",\"type\":\"output\"}],\"Top\":[]}"
  Connection Port : PMIOPort  Side=Left
  Out1 : Outport
  wires:
  Gain/1 -> Out1/1
  PS-Simulink Converter/1 -> Gain/1
  connections:
  Pressure Sensor (IL)/LConn1 -- Constant Volume Chamber (IL)/LConn1 -- Connection Port/RConn1
  PS-Simulink Converter/LConn1 -- Pressure Sensor (IL)/RConn1

== system Multibody_model_El_winch/Hydraulic System/DCV_cylinder/p_0 ==
  In1 : Inport
  Gain : Gain  Gain=10^5
  Pressure Source (IL) : fl_lib/Isothermal Liquid/Sources/Pressure Source (IL)  source_type=foundation.enum.constant_controlled.controlled  pressure_differential=0 MPa
      settings: InternalSimscapePortConfiguration="{\"Bottom\":[],\"Left\":[{\"id\":\"A\",\"label\":\"A\",\"type\":\"foundation.isothermal_liquid.isothermal_liquid\"},{\"id\":\"P\",\"label\":\"P\",\"type\":\"input\"}],\"Right\":[{\"id\":\"B\",\"label\":\"B\",\"type\":\"foundation.isothermal_liquid.isothermal_liquid\"}],\"Top\":[]}"
  Reservoir (IL) : fl_lib/Isothermal Liquid/Elements/Reservoir (IL)  reservoir_type=foundation.enum.constant_controlled.constant  pressure_spec=foundation.enum.pressure_spec.atmospheric  reservoir_pressure=0.101325 MPa
  Simulink-PS Converter : nesl_utility/Simulink-PS Converter  PhysicalDomain=network_engine_domain  SubClassName=ps_input  LeftPortType=input  RightPortType=output  PseudoPeriodic=off  Frequencies=[]  NoiseDistribution=none  NoiseParameters=[]  Unit=1  AffineConversion=off  FilteringAndDerivatives=provide  SimscapeFilterOrder=1  InputFilterTimeConstant=0.001  UdotUserProvided=0
  Connection Port : PMIOPort  Side=Left
  wires:
  In1/1 -> Gain/1
  Gain/1 -> Simulink-PS Converter/1
  connections:
  Reservoir (IL)/LConn1 -- Pressure Source (IL)/LConn1
  Simulink-PS Converter/RConn1 -- Pressure Source (IL)/LConn2
  Connection Port/RConn1 -- Pressure Source (IL)/RConn1

== system Multibody_model_El_winch/Hydraulic System/Pump/V_0 ==
  Constant Volume Chamber (IL) : fl_lib/Isothermal Liquid/Elements/Constant Volume Chamber (IL)  volume=1 l  p_I_specify=off  p_I_priority=High  p_I=0.101325 MPa  p_I_nominal_specify=off  p_I_nominal_unit=MPa  p_I_nominal_value=1
      settings: InternalSimscapePortConfiguration="{\"Bottom\":[],\"Left\":[{\"id\":\"A\",\"label\":\"A\",\"type\":\"foundation.isothermal_liquid.isothermal_liquid\"}],\"Right\":[],\"Top\":[]}"
  Gain : Gain  Gain=1/10^5
  PS-Simulink Converter : nesl_utility/PS-Simulink Converter  PhysicalDomain=network_engine_domain  SubClassName=ps_output  LeftPortType=input  RightPortType=output  PseudoPeriodic=off  Frequencies=[]  VectorFormat=inherit  Unit=inherit  AffineConversion=off
  Pressure Sensor (IL) : fl_lib/Isothermal Liquid/Sensors/Pressure Sensor (IL)  pressure_measure=foundation.enum.pressure_measure.gauge
      settings: InternalSimscapePortConfiguration="{\"Bottom\":[],\"Left\":[{\"id\":\"A\",\"label\":\"A\",\"type\":\"foundation.isothermal_liquid.isothermal_liquid\"}],\"Right\":[{\"id\":\"Pg\",\"label\":\"Pg\",\"type\":\"output\"}],\"Top\":[]}"
  Connection Port : PMIOPort  Side=Left
  Out1 : Outport
  wires:
  Gain/1 -> Out1/1
  PS-Simulink Converter/1 -> Gain/1
  connections:
  Pressure Sensor (IL)/LConn1 -- Constant Volume Chamber (IL)/LConn1 -- Connection Port/RConn1
  PS-Simulink Converter/LConn1 -- Pressure Sensor (IL)/RConn1

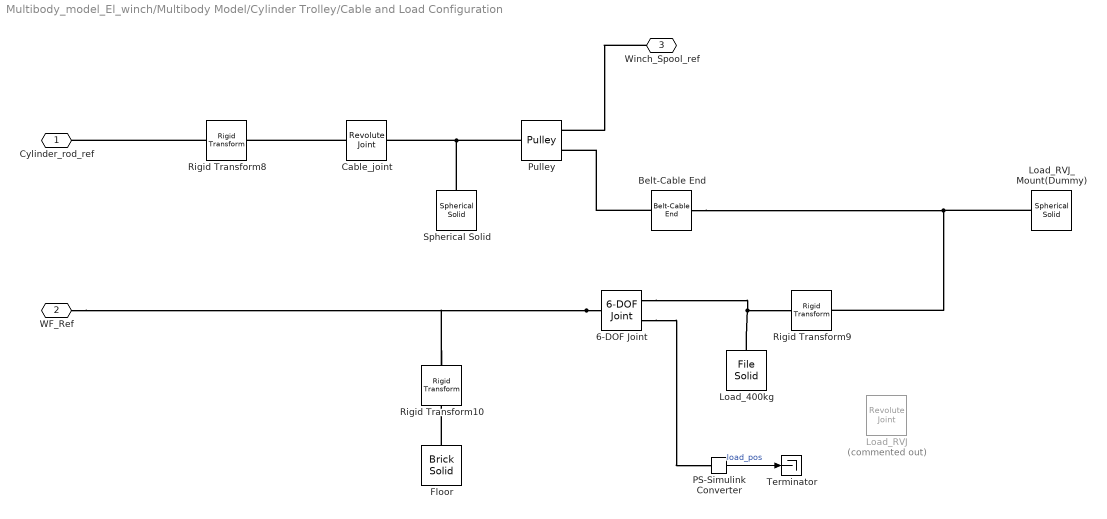
== system Multibody_model_El_winch/Multibody Model/Cylinder Trolley/Cable and Load Configuration ==
  6-DOF Joint : sm_lib/Joints/6-DOF Joint  JointMode=Normal  SenseConstraintForce=off  SenseConstraintForceX=off  SenseConstraintForceY=off  SenseConstraintForceZ=off  SenseConstraintTorque=off  SenseConstraintTorqueX=off  SenseConstraintTorqueY=off  SenseConstraintTorqueZ=off  SenseTotalForce=off  SenseTotalForceX=off  SenseTotalForceY=off  SenseTotalForceZ=off  SenseTotalTorque=off  SenseTotalTorqueX=off  SenseTotalTorqueY=off  SenseTotalTorqueZ=off  CompositeWrenchDir=FollowerOnBase  CompositeWrenchFrame=BaseFrame  PxEquilibriumPosition=0  PxEquilibriumPositionUnits=m  PxSpringStiffness=0  PxSpringStiffnessUnits=N/m  PxDampingCoefficient=0  PxDampingCoefficientUnits=N/(m/s)  PxTorqueActuationMode=NoTorque  PxMotionActuationMode=ComputedMotion  PxSensePosition=off  PxSenseVelocity=off  PxSenseAcceleration=off  PxSenseTorqueForce=off  PxSenseLowerLimitTorqueForce=off  PxSenseUpperLimitTorqueForce=off  PxLowerLimitSpecify=off  PxLowerLimitBound=0  PxLowerLimitBoundUnits=m  PxLowerLimitStiffness=1e6  PxLowerLimitStiffnessUnits=N/m  PxLowerLimitDamping=1e3  PxLowerLimitDampingUnits=N/(m/s)  PxLowerLimitTransitionRegionWidth=1e-4  PxLowerLimitTransitionRegionWidthUnits=m  PxUpperLimitSpecify=off  PxUpperLimitBound=1  PxUpperLimitBoundUnits=m  PxUpperLimitStiffness=1e6  PxUpperLimitStiffnessUnits=N/m  PxUpperLimitDamping=1e3  PxUpperLimitDampingUnits=N/(m/s)  PxUpperLimitTransitionRegionWidth=1e-4  PxUpperLimitTransitionRegionWidthUnits=m  PxPositionTargetSpecify=on  PxPositionTargetPriority=High  PxPositionTargetValue=-877  PxPositionTargetValueUnits=mm  PxVelocityTargetSpecify=off  PxVelocityTargetPriority=High  PxVelocityTargetValue=0  PxVelocityTargetValueUnits=m/s  PyEquilibriumPosition=0  PyEquilibriumPositionUnits=m  PySpringStiffness=0  PySpringStiffnessUnits=N/m  PyDampingCoefficient=0  PyDampingCoefficientUnits=N/(m/s)  PyTorqueActuationMode=NoTorque  PyMotionActuationMode=ComputedMotion  PySensePosition=off  PySenseVelocity=off  PySenseAcceleration=off  PySenseTorqueForce=off  PySenseLowerLimitTorqueForce=off  PySenseUpperLimitTorqueForce=off  PyLowerLimitSpecify=off  PyLowerLimitBound=-1  PyLowerLimitBoundUnits=m  PyLowerLimitStiffness=1e6  PyLowerLimitStiffnessUnits=N/m  PyLowerLimitDamping=1e3  PyLowerLimitDampingUnits=N/(m/s)  PyLowerLimitTransitionRegionWidth=1e-4  PyLowerLimitTransitionRegionWidthUnits=m  PyUpperLimitSpecify=off  PyUpperLimitBound=1  PyUpperLimitBoundUnits=m  PyUpperLimitStiffness=1e6  PyUpperLimitStiffnessUnits=N/m  PyUpperLimitDamping=1e3  PyUpperLimitDampingUnits=N/(m/s)  PyUpperLimitTransitionRegionWidth=1e-4  PyUpperLimitTransitionRegionWidthUnits=m  PyPositionTargetSpecify=on  PyPositionTargetPriority=High  PyPositionTargetValue=190+120  PyPositionTargetValueUnits=mm  PyVelocityTargetSpecify=off  PyVelocityTargetPriority=High  PyVelocityTargetValue=0  PyVelocityTargetValueUnits=m/s  PzEquilibriumPosition=0  PzEquilibriumPositionUnits=m  PzSpringStiffness=0  PzSpringStiffnessUnits=N/m  PzDampingCoefficient=0  PzDampingCoefficientUnits=N/(m/s)  PzTorqueActuationMode=NoTorque  PzMotionActuationMode=ComputedMotion  PzSensePosition=on  PzSenseVelocity=off  PzSenseAcceleration=off  PzSenseTorqueForce=off  PzSenseLowerLimitTorqueForce=off  PzSenseUpperLimitTorqueForce=off  PzLowerLimitSpecify=off  PzLowerLimitBound=-1  PzLowerLimitBoundUnits=m  PzLowerLimitStiffness=1e6  PzLowerLimitStiffnessUnits=N/m  PzLowerLimitDamping=1e3  PzLowerLimitDampingUnits=N/(m/s)  PzLowerLimitTransitionRegionWidth=1e-4  PzLowerLimitTransitionRegionWidthUnits=m  PzUpperLimitSpecify=off  PzUpperLimitBound=1  PzUpperLimitBoundUnits=m  PzUpperLimitStiffness=1e6  PzUpperLimitStiffnessUnits=N/m  PzUpperLimitDamping=1e3  PzUpperLimitDampingUnits=N/(m/s)  PzUpperLimitTransitionRegionWidth=1e-4  PzUpperLimitTransitionRegionWidthUnits=m  PzPositionTargetSpecify=on  PzPositionTargetPriority=High  PzPositionTargetValue=120  PzPositionTargetValueUnits=mm  PzVelocityTargetSpecify=off  PzVelocityTargetPriority=High  PzVelocityTargetValue=0  PzVelocityTargetValueUnits=m/s  SphEqPosRotationMethod=None  SphEqPosRotationAngleUnits=deg  SphEqPosRotationStandardAxis=+Z  SphEqPosRotationAngle=0.0  SphEqPosRotationArbitraryAxis=[0 0 1]  SphEqPosFollAlignAxisA=+X  SphEqPosBaseAlignAxisA=+Y  SphEqPosFollAlignAxisB=+Y  SphEqPosBaseAlignAxisB=+Z  SphEqPosRotationSequenceAxes=FollowerAxes  SphEqPosRotationSequence=XYX  SphEqPosRotationSequenceAngles=[0 0 0]  SphEqPosRotationSequenceAnglesUnits=deg  SphEqPosRotationMatrix=[1 0 0; 0 1 0; 0 0 1]  SphEqPosQuaternion=[1 0 0 0]  SphSpringStiffness=0  SphSpringStiffnessUnits=N*m/deg  SphDampingCoefficient=0  SphDampingCoefficientUnits=N*m/(deg/s)  SphActuateTorqueX=off  SphActuateTorqueY=off  SphActuateTorqueZ=off  SphActuateTorque=off  SphTorqueActuationMode=NoTorque  SphMotionActuationMode=ComputedMotion  SphActuationFrame=BaseFrame  SphSensePosition=off  SphSenseVelocityX=off  SphSenseVelocityY=off  SphSenseVelocityZ=off  SphSenseVelocity=off  SphSenseAccelerationX=off  SphSenseAccelerationY=off  SphSenseAccelerationZ=off  SphSenseAcceleration=off  SphSenseTorqueX=off  SphSenseTorqueY=off  SphSenseTorqueZ=off  SphSenseTorqueForce=off  SphSenseLowerLimitTorqueMag=off  SphSenseUpperLimitTorqueMag=off  SphSensingFrame=BaseFrame  SphLowerLimitSpecify=off  SphLowerLimitBound=15  SphLowerLimitBoundUnits=deg  SphLowerLimitStiffness=1e4  SphLowerLimitStiffnessUnits=N*m/deg  SphLowerLimitDamping=10  SphLowerLimitDampingUnits=N*m/(deg/s)  SphLowerLimitTransitionRegionWidth=0.1  SphLowerLimitTransitionRegionWidthUnits=deg  SphUpperLimitSpecify=off  SphUpperLimitBound=45  SphUpperLimitBoundUnits=deg  SphUpperLimitStiffness=1e4  SphUpperLimitStiffnessUnits=N*m/deg  SphUpperLimitDamping=10  SphUpperLimitDampingUnits=N*m/(deg/s)  SphUpperLimitTransitionRegionWidth=0.1  SphUpperLimitTransitionRegionWidthUnits=deg  SphPositionTargetRotationMethod=None  SphPositionTargetRotationAngleUnits=deg  SphPositionTargetRotationStandardAxis=+Z  SphPositionTargetRotationAngle=0.0  SphPositionTargetRotationArbitraryAxis=[0 0 1]  SphPositionTargetFollAlignAxisA=+X  SphPositionTargetBaseAlignAxisA=+Y  SphPositionTargetFollAlignAxisB=+Y  SphPositionTargetBaseAlignAxisB=+Z  SphPositionTargetRotationSequenceAxes=FollowerAxes  SphPositionTargetRotationSequence=XYX  SphPositionTargetRotationSequenceAngles=[0 0 0]  SphPositionTargetRotationSequenceAnglesUnits=deg  SphPositionTargetRotationMatrix=[1 0 0; 0 1 0; 0 0 1]  SphPositionTargetQuaternion=[1 0 0 0]  SphPositionTargetSpecify=off  SphPositionTargetPriority=High  SphVelocityTargetValue=[0 0 0]  SphVelocityTargetValueUnits=deg/s  SphVelocityTargetSpecify=off  SphVelocityTargetPriority=High  SphVelocityTargetInFollowerFrame=on
  Belt-Cable End : sm_lib/Belts and Cables/Belt-Cable End
  Cable_joint : sm_lib/Joints/Revolute Joint  JointMode=Normal  SenseConstraintForce=off  SenseConstraintForceX=off  SenseConstraintForceY=off  SenseConstraintForceZ=off  SenseConstraintTorque=off  SenseConstraintTorqueX=off  SenseConstraintTorqueY=off  SenseConstraintTorqueZ=off  SenseTotalForce=off  SenseTotalForceX=off  SenseTotalForceY=off  SenseTotalForceZ=off  SenseTotalTorque=off  SenseTotalTorqueX=off  SenseTotalTorqueY=off  SenseTotalTorqueZ=off  CompositeWrenchDir=FollowerOnBase  CompositeWrenchFrame=BaseFrame  EquilibriumPosition=0  EquilibriumPositionUnits=deg  SpringStiffness=0  SpringStiffnessUnits=N*m/deg  DampingCoefficient=0  DampingCoefficientUnits=N*m/(deg/s)  TorqueActuationMode=NoTorque  MotionActuationMode=ComputedMotion  SensePosition=off  SenseVelocity=off  SenseAcceleration=off  SenseTorqueForce=off  SenseLowerLimitTorqueForce=off  SenseUpperLimitTorqueForce=off  LowerLimitSpecify=off  LowerLimitBound=-90  LowerLimitBoundUnits=deg  LowerLimitStiffness=1e4  LowerLimitStiffnessUnits=N*m/deg  LowerLimitDamping=10  LowerLimitDampingUnits=N*m/(deg/s)  LowerLimitTransitionRegionWidth=0.1  LowerLimitTransitionRegionWidthUnits=deg  UpperLimitSpecify=off  UpperLimitBound=90  UpperLimitBoundUnits=deg  UpperLimitStiffness=1e4  UpperLimitStiffnessUnits=N*m/deg  UpperLimitDamping=10  UpperLimitDampingUnits=N*m/(deg/s)  UpperLimitTransitionRegionWidth=0.1  UpperLimitTransitionRegionWidthUnits=deg  PositionTargetSpecify=off  PositionTargetPriority=High  PositionTargetValue=0  PositionTargetValueUnits=deg  VelocityTargetSpecify=off  VelocityTargetPriority=High  VelocityTargetValue=0  VelocityTargetValueUnits=deg/s
  Floor : sm_lib/Body Elements/Brick Solid  GraphicAmbientColor=[0.15 0.15 0.15 1.0]  BasedOnType=Density  BrickDimensions=[3 1 0.1]  BrickDimensionsUnits=m  CenterOfMass=[0 0 0]  CenterOfMassUnits=m  GraphicDiffuseColor=[1.0 1.0 1.0]  Density=1000  DensityUnits=kg/m^3  DoExposeReferenceFrame=on  GraphicEmissiveColor=[0.0 0.0 0.0 1.0]  ExportEntireGeometry=off  SerializedFrames=<Frames/>  MarkerShape=Sphere  MarkerSize=10  GraphicType=FromGeometry  InertiaType=Custom  Mass=1  MassUnits=kg  MomentsOfInertia=[1 1 1]  MomentsOfInertiaUnits=kg*m^2  GraphicOpacity=1.0  ProductsOfInertia=[0 0 0]  ProductsOfInertiaUnits=kg*m^2  GraphicShininess=75  GraphicSpecularColor=[0.5 0.5 0.5 1.0]  GraphicVisPropType=SimpleVisualProperties
  Load_400kg : sm_lib/Body Elements/File Solid  ExtGeomFileName=.\Parts_and_stl\Load.STL  UnitType=Custom  ExtGeomFileUnits=mm  StepReaderType=HEX  ExportConvexHullGeometry=off  InertiaType=Custom  Mass=1000  MassUnits=kg  CenterOfMass=[0 0 0]  CenterOfMassUnits=m  MomentsOfInertia=[115.546313 927.95 846.2595]  MomentsOfInertiaUnits=kg*m^2  ProductsOfInertia=[0 0 0]  ProductsOfInertiaUnits=kg*m^2  BasedOnType=DensityFromFile  Density=1000  DensityUnits=kg/m^3  DoExposeReferenceFrame=on  SerializedFrames=<Frames/>  GraphicType=FromGeometry  MarkerShape=Sphere  MarkerSize=10  GraphicVisPropType=SimpleVisualProperties  GraphicDiffuseColor=[0.5 0.5 0.5]  GraphicSpecularColor=[0.5 0.5 0.5 1.0]  GraphicAmbientColor=[0.15 0.15 0.15 1.0]  GraphicEmissiveColor=[0.0 0.0 0.0 1.0]  GraphicShininess=75  GraphicOpacity=1.0
  Load_RVJ : sm_lib/Joints/Revolute Joint  Commented=on  JointMode=Normal  SenseConstraintForce=off  SenseConstraintForceX=off  SenseConstraintForceY=off  SenseConstraintForceZ=off  SenseConstraintTorque=off  SenseConstraintTorqueX=off  SenseConstraintTorqueY=off  SenseConstraintTorqueZ=off  SenseTotalForce=off  SenseTotalForceX=off  SenseTotalForceY=off  SenseTotalForceZ=off  SenseTotalTorque=off  SenseTotalTorqueX=off  SenseTotalTorqueY=off  SenseTotalTorqueZ=off  CompositeWrenchDir=FollowerOnBase  CompositeWrenchFrame=BaseFrame  EquilibriumPosition=0  EquilibriumPositionUnits=deg  SpringStiffness=0  SpringStiffnessUnits=N*m/deg  DampingCoefficient=0  DampingCoefficientUnits=N*m/(deg/s)  TorqueActuationMode=NoTorque  MotionActuationMode=ComputedMotion  SensePosition=off  SenseVelocity=off  SenseAcceleration=off  SenseTorqueForce=off  SenseLowerLimitTorqueForce=off  SenseUpperLimitTorqueForce=off  LowerLimitSpecify=off  LowerLimitBound=-90  LowerLimitBoundUnits=deg  LowerLimitStiffness=1e4  LowerLimitStiffnessUnits=N*m/deg  LowerLimitDamping=10  LowerLimitDampingUnits=N*m/(deg/s)  LowerLimitTransitionRegionWidth=0.1  LowerLimitTransitionRegionWidthUnits=deg  UpperLimitSpecify=off  UpperLimitBound=90  UpperLimitBoundUnits=deg  UpperLimitStiffness=1e4  UpperLimitStiffnessUnits=N*m/deg  UpperLimitDamping=10  UpperLimitDampingUnits=N*m/(deg/s)  UpperLimitTransitionRegionWidth=0.1  UpperLimitTransitionRegionWidthUnits=deg  PositionTargetSpecify=off  PositionTargetPriority=High  PositionTargetValue=0  PositionTargetValueUnits=deg  VelocityTargetSpecify=off  VelocityTargetPriority=High  VelocityTargetValue=0  VelocityTargetValueUnits=deg/s
  Load_RVJ_Mount(Dummy) : sm_lib/Body Elements/Spherical Solid  GraphicAmbientColor=[0.15 0.15 0.15 1.0]  BasedOnType=Density  CenterOfMass=[0 0 0]  CenterOfMassUnits=m  GraphicDiffuseColor=[0.5 0.5 0.5]  Density=1000  DensityUnits=kg/m^3  DoExposeReferenceFrame=on  GraphicEmissiveColor=[0.0 0.0 0.0 1.0]  ExportEntireGeometry=off  SerializedExposedGeometries=<ExposedGeometries/>  SerializedFrames=<Frames/>  MarkerShape=Sphere  MarkerSize=10  GraphicType=FromGeometry  InertiaType=Custom  Mass=1  MassUnits=kg  MomentsOfInertia=[1 1 1]  MomentsOfInertiaUnits=kg*m^2  GraphicOpacity=1.0  ProductsOfInertia=[0 0 0]  ProductsOfInertiaUnits=kg*m^2  GraphicShininess=75  GraphicSpecularColor=[0.5 0.5 0.5 1.0]  SphereRadius=2  SphereRadiusUnits=cm  GraphicVisPropType=SimpleVisualProperties
  PS-Simulink Converter : nesl_utility/PS-Simulink Converter  PhysicalDomain=network_engine_domain  SubClassName=ps_output  LeftPortType=input  RightPortType=output  PseudoPeriodic=off  Frequencies=[]  VectorFormat=inherit  Unit=inherit  AffineConversion=off
  Pulley : sm_lib/Belts and Cables/Pulley  PitchRadius=85/2  PitchRadiusUnits=mm  InitialWrapAngleLowerBound=0  InitialWrapAngleLowerBoundUnits=deg  SenseWrapAngle=off  SensePulleyAngleA=off  SensePulleyAngleB=off  SenseFleetAngleA=off  SenseFleetAngleB=off
  Rigid Transform10 : sm_lib/Frames and Transforms/Rigid Transform  TranslationMethod=Cartesian  TranslationStandardOffset=0  TranslationStandardOffsetUnits=m  TranslationStandardAxis=+Z  TranslationCartesianOffset=[-1100 290 -70]  TranslationCartesianOffsetUnits=mm  TranslationROffset=0  TranslationROffsetUnits=m  TranslationZOffset=0  TranslationZOffsetUnits=m  TranslationThetaOffset=0  TranslationThetaOffsetUnits=deg  RotationMethod=None  RotationAngleUnits=deg  RotationStandardAxis=+Z  RotationAngle=0.0  RotationArbitraryAxis=[0 0 1]  FollAlignAxisA=+X  BaseAlignAxisA=+Y  FollAlignAxisB=+Y  BaseAlignAxisB=+Z  RotationSequenceAxes=FollowerAxes  RotationSequence=XYX  RotationSequenceAngles=[0 0 0]  RotationSequenceAnglesUnits=deg  RotationMatrix=[1 0 0; 0 1 0; 0 0 1]  Quaternion=[1 0 0 0]
  Rigid Transform8 : sm_lib/Frames and Transforms/Rigid Transform  TranslationMethod=Cartesian  TranslationStandardOffset=0  TranslationStandardOffsetUnits=m  TranslationStandardAxis=+Z  TranslationCartesianOffset=[115 0 0]  TranslationCartesianOffsetUnits=mm  TranslationROffset=0  TranslationROffsetUnits=m  TranslationZOffset=0  TranslationZOffsetUnits=m  TranslationThetaOffset=0  TranslationThetaOffsetUnits=deg  RotationMethod=None  RotationAngleUnits=deg  RotationStandardAxis=+Z  RotationAngle=0.0  RotationArbitraryAxis=[0 0 1]  FollAlignAxisA=+X  BaseAlignAxisA=+Y  FollAlignAxisB=+Y  BaseAlignAxisB=+Z  RotationSequenceAxes=FollowerAxes  RotationSequence=XYX  RotationSequenceAngles=[0 0 0]  RotationSequenceAnglesUnits=deg  RotationMatrix=[1 0 0; 0 1 0; 0 0 1]  Quaternion=[1 0 0 0]
  Rigid Transform9 : sm_lib/Frames and Transforms/Rigid Transform  TranslationMethod=Cartesian  TranslationStandardOffset=0  TranslationStandardOffsetUnits=m  TranslationStandardAxis=+Z  TranslationCartesianOffset=[0 0 120]  TranslationCartesianOffsetUnits=mm  TranslationROffset=0  TranslationROffsetUnits=m  TranslationZOffset=0  TranslationZOffsetUnits=m  TranslationThetaOffset=0  TranslationThetaOffsetUnits=deg  RotationMethod=RotationSequence  RotationAngleUnits=deg  RotationStandardAxis=+Z  RotationAngle=0.0  RotationArbitraryAxis=[0 0 1]  FollAlignAxisA=+X  BaseAlignAxisA=+Y  FollAlignAxisB=+Y  BaseAlignAxisB=+Z  RotationSequenceAxes=FollowerAxes  RotationSequence=XYZ  RotationSequenceAngles=[90 0 0]  RotationSequenceAnglesUnits=deg  RotationMatrix=[1 0 0; 0 1 0; 0 0 1]  Quaternion=[1 0 0 0]
  Spherical Solid : sm_lib/Body Elements/Spherical Solid  GraphicAmbientColor=[0.15 0.15 0.15 1.0]  BasedOnType=Density  CenterOfMass=[0 0 0]  CenterOfMassUnits=m  GraphicDiffuseColor=[0.5 0.5 0.5]  Density=1000  DensityUnits=kg/m^3  DoExposeReferenceFrame=on  GraphicEmissiveColor=[0.0 0.0 0.0 1.0]  ExportEntireGeometry=off  SerializedExposedGeometries=<ExposedGeometries/>  SerializedFrames=<Frames/>  MarkerShape=Sphere  MarkerSize=10  GraphicType=FromGeometry  InertiaType=Custom  Mass=1  MassUnits=kg  MomentsOfInertia=[1 1 1]  MomentsOfInertiaUnits=kg*m^2  GraphicOpacity=1.0  ProductsOfInertia=[0 0 0]  ProductsOfInertiaUnits=kg*m^2  GraphicShininess=75  GraphicSpecularColor=[0.5 0.5 0.5 1.0]  SphereRadius=0.01  SphereRadiusUnits=m  GraphicVisPropType=SimpleVisualProperties
  Terminator : Terminator
  Cylinder_rod_ref : PMIOPort  Side=Left
  WF_Ref : PMIOPort  Port=2  Side=Left
  Winch_Spool_ref : PMIOPort  Port=3  Side=Left
  wires:
  PS-Simulink Converter/1 -> Terminator/1  "load_pos"
  connections:
  Belt-Cable End/RConn1 -- Pulley/RConn2
  6-DOF Joint/RConn1 -- Load_400kg/RConn1 -- Rigid Transform9/LConn1
  Pulley/LConn1 -- Spherical Solid/RConn1 -- Cable_joint/RConn1
  Floor/RConn1 -- Rigid Transform10/RConn1
  6-DOF Joint/LConn1 -- WF_Ref/RConn1 -- Rigid Transform10/LConn1
  Cable_joint/LConn1 -- Rigid Transform8/RConn1
  Rigid Transform8/LConn1 -- Cylinder_rod_ref/RConn1
  Belt-Cable End/LConn1 -- Rigid Transform9/RConn1 -- Load_RVJ_Mount(Dummy)/RConn1
  Winch_Spool_ref/RConn1 -- Pulley/RConn1
  6-DOF Joint/RConn2 -- PS-Simulink Converter/LConn1

== system Multibody_model_El_winch/Electrical Winch/Current Controller and Flux Estimator/IM/Electromagnetic Torque ==
  note: lecture 5 equation 26
  i_s^s : Inport
  psi_R^s : Inport  Port=2
  Complex to Real-Imag : ComplexToRealImag  Output=Imag
  Gain : Gain  Gain=3*np/2
  Product : Product
  conj : Math  Operator=conj
  T_em : Outport
  wires:
  psi_R^s/1 -> conj/1
  i_s^s/1 -> Product/1
  conj/1 -> Product/2
  Product/1 -> Complex to Real-Imag/1
  Complex to Real-Imag/1 -> Gain/1
  Gain/1 -> T_em/1

== system Multibody_model_El_winch/Electrical Winch/Current Controller and Flux Estimator/IM/Flux Equations ==
  note: lecture 5 eq. 16 and 17
  psi_s^s : Inport
  psi_R^s : Inport  Port=2
  Constant : Constant  Value=L_M_hat
  Eq(16) : Gain  Gain=1/L_sig_hat
  Gain1 : Gain  Gain=1/L_M_hat
  Subtract : Sum  Inputs=+-
  Sum : Sum  Inputs=|+-
  i_s^s : Outport
  i_R^s : Outport  Port=2
  I_M : Outport  Port=3
  wires:
  psi_s^s/1 -> Sum/1
  Sum/1 -> Eq(16)/1  "i_R = I_M^s - i_s^s"
  psi_R^s/1 -> Gain1/1, Sum/2
  Subtract/1 -> i_R^s/1
  Eq(16)/1 -> i_s^s/1, Subtract/2
  Gain1/1 -> Subtract/1, I_M/1

== system Multibody_model_El_winch/Electrical Winch/Current Controller and Flux Estimator/IM/Voltage Equations ==
  v_s^s : Inport
  i_s^s : Inport  Port=2
  w_r : Inport  Port=3
  i_R^s : Inport  Port=4
  Gain : Gain  Gain=R_s
  Gain1 : Gain  Gain=R_R
  Gain2 : Gain  Gain=1j
  Integrator (Complex Signal) : Subsystem
      mask Display: disp('1/s');
  Integrator (Complex Signal)1 : Subsystem
      mask Display: disp('1/s');
  Product : Product  RndMeth=Zero
  Sum1 : Sum  Inputs=|+-
  Sum2 : Sum  Inputs=|-+
  psi_s^s : Outport
  psi_R^s : Outport  Port=2
  wires:
  w_r/1 -> Product/2
  Gain2/1 -> Product/1
  Integrator (Complex Signal)1/1(y) -> Gain2/1, psi_R^s/1
  Integrator (Complex Signal)/1(y) -> psi_s^s/1
  Gain/1 -> Sum1/2
  Sum1/1 -> Integrator (Complex Signal)/1(u)  "dpsi_s^s"
  i_s^s/1 -> Gain/1
  v_s^s/1 -> Sum1/1
  Product/1 -> Sum2/2  "j *w_r*psi_R^s"
  i_R^s/1 -> Gain1/1
  Gain1/1 -> Sum2/1
  Sum2/1 -> Integrator (Complex Signal)1/1(u)  "dpsi_s^s"

== system Multibody_model_El_winch/Electrical Winch/Current Controller and Flux Estimator/IM/abc->alphabeta ==
  vs_abc : Inport
  Fcn : Fcn  Expr=2/3*(u(1)-0.5*u(2)-0.5*u(3))
  Fcn1 : Fcn  Expr=sqrt(3)/3*(u(2)-u(3))
  Real-Imag to Complex : RealImagToComplex
  v_s^s : Outport
  wires:
  Real-Imag to Complex/1 -> v_s^s/1
  Fcn1/1 -> Real-Imag to Complex/2  "beta"
  Fcn/1 -> Real-Imag to Complex/1  "alpha"
  vs_abc/1 -> Fcn/1, Fcn1/1
